simulink model "HQEV_MiL_20160830_integrate_r2017a"  (Simulink 8.9)
settings: Solver=FixedStepDiscrete  StartTime=0.0  StopTime=inf  FixedStep=0.01  RelTol=1e-3  EnableMultiTasking=on
PostLoadFcn:
  | , if any(exist('dsrtsu_mdlpostloadfcn', 'file') == [2, 3, 6]), try dsrtsu_mdlpostloadfcn('Execute', bdroot); catch fprintf('Error in PostLoadFcn (dsrtsu_mdlpostloadfcn) for model "%s":\n %s\n', bdroot, lasterr); end, end,
values from neighbouring files (symbols this model uses):
  Bat_C_Ah = 36    [parameter_V1.mat]
  Bat_ocv_xIndex = [5 10 20 30 40 50 60 70 80 90 95]    [parameter_V1.mat]
  Bat_ocv_z = [329 332 340 345 347 351 358 372 377 386 391]    [parameter_V1.mat]
  Bat_R_ohm_z = [4.41 3.46 1.57 1.07 0.76 0.63 0.55 0.44 0.41 0.4 0.4 3.14 ... (66 elements, 11x6)]    [parameter_V1.mat]
  Bat_SOC_Init = 90    [parameter_V1.mat]
  Env_hum_pct_Ambient = 30    [parameter_V1.mat]
  Env_Slope_deg = 0    [parameter_V1.mat]
  Env_Temp_degC_Ambient = 25    [parameter_V1.mat]
  Env_v_kmph_HWind = 0    [parameter_V1.mat]
  Reducer_F_i = 7.23    [parameter_V1.mat]
  Reducer_R_i = 7.23    [parameter_V1.mat]
  Veh =     [parameter_V1.mat]
  Veh_A_m2_Fr = 2.246    [parameter_V1.mat]
  Veh_F_Brake =     [parameter_V1.mat]
  Veh_fac_AirDrag = 0.326    [parameter_V1.mat]
  Veh_fac_WhDragFrict_0 = 0.011    [parameter_V1.mat]
  Veh_g_mps2_C = 9.81    [parameter_V1.mat]
  Veh_GainBrake =     [parameter_V1.mat]
  Veh_h_m_COGHigh = 0.5    [parameter_V1.mat]
  Veh_J_kgm2_Wh = 1.3635    [parameter_V1.mat]
  Veh_L_m_AxlBas = 2.63    [parameter_V1.mat]
  Veh_M_kg = 1427    [parameter_V1.mat]
  Veh_mu_Brake = 0.4    [parameter_V1.mat]
  Veh_mu_Tyre =     [parameter_V1.mat]
  Veh_num_FrictPair = 8    [parameter_V1.mat]
  Veh_pct_Brk = 70    [parameter_V1.mat]
  Veh_r_dyn =     [parameter_V1.mat]
  Veh_r_m_BrkDisk = 0.136    [parameter_V1.mat]
  Veh_rho_kgpm3_Air = 1.2258    [parameter_V1.mat]
undefined symbols (not defined in the file or in its folder): DiscIntNeverNeededParam, p_bool_False_M, p_bool_True_M
libraries: BaseOperationLib_Browser x38, simulink x8, DTQC_lib x1, ERR_lib x1, MQM_lib x1, PTCL_lib x1, PUD_lib x1, TQD_lib x1, TQR_lib x1, VMM_lib x1, ACCA_lib x1, BBCA_lib x1
(part 5 of 15)

== system HQEV_MiL_20160830_integrate_r2017a/MiL/Test_Integration/ESP/Subsystem/ABS ==
  In1 : Inport
  Bus Selector : BusSelector  OutputSignals=Vehicle.v_Veh
  Bus Selector1 : BusSelector  OutputSignals=Drv.signal1.BrkPed_pct
  Bus Selector2 : BusSelector  OutputSignals=IO.ABS_ErrorStatus,IO.ABS_Intervention,IO.ASR1_ASRErrorStatus,IO.ASR1_ASRIntervention,IO.ESP_ErrorStatus,IO.ESP_Intervention
  Constant{,1..3,10..11} (6 alike) : Constant  Value=0
  Lookup Table : Lookup  InputValues=[0 100]  Table=[0 200]
  Checksum_ABS_1 : Outport
  WheelSpeed_FL : Outport  Port=2
  WheelSpeed_FR : Outport  Port=3
  ABS_VehicleSpeed : Outport  Port=4
  LiveCounter_ABS_1 : Outport  Port=5
  Checksum_ABS_2 : Outport  Port=6
  WheelSpeed_RL : Outport  Port=7
  WheelSpeed_RR : Outport  Port=8
  ABS_MasterCylinderPressure : Outport  Port=9
  LiveCounter_ABS_2 : Outport  Port=10
  ABS_ErrorStatus : Outport  Port=11
  ABS_Intervention : Outport  Port=12
  ASR_ErrorStatus : Outport  Port=13
  ASR_Intervention : Outport  Port=14
  ESP_ErrorStatus : Outport  Port=15
  ESP_Intervention : Outport  Port=16
  HHC_Status : Outport  Port=17
  HHC_Available : Outport  Port=18
  wires:
  Constant/1 -> Checksum_ABS_1/1
  In1/1 -> Bus Selector/1, Bus Selector2/1, Bus Selector1/1
  Bus Selector/1 -> WheelSpeed_FL/1, WheelSpeed_FR/1, ABS_VehicleSpeed/1, WheelSpeed_RL/1, WheelSpeed_RR/1  "<v_Veh>"
  Constant1/1 -> LiveCounter_ABS_1/1
  Constant2/1 -> Checksum_ABS_2/1
  Bus Selector1/1 -> Lookup Table/1  "<BrkPed_pct>"
  Lookup Table/1 -> ABS_MasterCylinderPressure/1
  Constant3/1 -> LiveCounter_ABS_2/1
  Bus Selector2/1 -> ABS_ErrorStatus/1  "<ABS_ErrorStatus>"
  Bus Selector2/2 -> ABS_Intervention/1  "<ABS_Intervention>"
  Bus Selector2/3 -> ASR_ErrorStatus/1  "<ASR1_ASRErrorStatus>"
  Bus Selector2/4 -> ASR_Intervention/1  "<ASR1_ASRIntervention>"
  Bus Selector2/5 -> ESP_ErrorStatus/1  "<ESP_ErrorStatus>"
  Bus Selector2/6 -> ESP_Intervention/1  "<ESP_Intervention>"
  Constant10/1 -> HHC_Status/1
  Constant11/1 -> HHC_Available/1

== system HQEV_MiL_20160830_integrate_r2017a/MiL/Test_Integration/ESP/Subsystem/ASR ==
  In1 : Inport
  Bus Selector2 : BusSelector  OutputSignals=IO.ASR_TorqueReductionFast,IO.MSR_TorqueIncrease,IO.ASR_StatusTRFast,IO.MSR_StatusTI
  Constant : Constant  Value=0
  Constant3 : Constant  Value=0
  Checksum_ASR_1 : Outport
  ASR_TorqueReductionFast : Outport  Port=2
  MSR_TorqueIncrease : Outport  Port=3
  LiveCounter_ASR_1 : Outport  Port=4
  ASR_StatusTRFast : Outport  Port=5
  MSR_StatusTI : Outport  Port=6
  wires:
  In1/1 -> Bus Selector2/1
  Constant/1 -> Checksum_ASR_1/1
  Bus Selector2/1 -> ASR_TorqueReductionFast/1  "<ASR_TorqueReductionFast>"
  Bus Selector2/2 -> MSR_TorqueIncrease/1  "<MSR_TorqueIncrease>"
  Constant3/1 -> LiveCounter_ASR_1/1
  Bus Selector2/3 -> ASR_StatusTRFast/1  "<ASR_StatusTRFast>"
  Bus Selector2/4 -> MSR_StatusTI/1  "<MSR_StatusTI>"

== system HQEV_MiL_20160830_integrate_r2017a/MiL/Test_Integration/ESP/Subsystem/ASR2 ==
  In1 : Inport
  Bus Selector51 : BusSelector  OutputSignals=IO
  Bus Selector52 : BusSelector  OutputSignals=ASR2TrqRdctFastASR2,ASR2TrqIncrsMSR2,ASR2StTRFastASR2,ASR2StTIMSR2,ABS6RegenTrqReq,ABS6StRegenTrqReq
  ASR2TrqRdctFastASR2 : Outport
  ASR2TrqIncrsMSR2 : Outport  Port=2
  ASR2StTRFastASR2 : Outport  Port=3
  ASR2StTIMSR2 : Outport  Port=4
  ABS6RegenTrqReq : Outport  Port=5
  ABS6StRegenTrqReq : Outport  Port=6
  wires:
  Bus Selector51/1 -> Bus Selector52/1  "<IO>"
  In1/1 -> Bus Selector51/1
  Bus Selector52/1 -> ASR2TrqRdctFastASR2/1  "<ASR2TrqRdctFastASR2>"
  Bus Selector52/2 -> ASR2TrqIncrsMSR2/1  "<ASR2TrqIncrsMSR2>"
  Bus Selector52/3 -> ASR2StTRFastASR2/1  "<ASR2StTRFastASR2>"
  Bus Selector52/4 -> ASR2StTIMSR2/1  "<ASR2StTIMSR2>"
  Bus Selector52/5 -> ABS6RegenTrqReq/1  "<ABS6RegenTrqReq>"
  Bus Selector52/6 -> ABS6StRegenTrqReq/1  "<ABS6StRegenTrqReq>"

== system HQEV_MiL_20160830_integrate_r2017a/MiL/Test_Integration/ESP/Subsystem/EPB ==
  In1 : Inport
  Constant{,1..3} (4 alike) : Constant  Value=0
  Terminator : Terminator
  Checksum_EPB_1 : Outport
  LiveCounter_EPB_1 : Outport  Port=2
  EPB_Status : Outport  Port=3
  EPB_ErrorStatus : Outport  Port=4
  wires:
  Constant/1 -> Checksum_EPB_1/1
  Constant1/1 -> LiveCounter_EPB_1/1
  Constant2/1 -> EPB_Status/1
  Constant3/1 -> EPB_ErrorStatus/1
  In1/1 -> Terminator/1

== system HQEV_MiL_20160830_integrate_r2017a/MiL/Test_Integration/ESP/Subsystem/YRS ==
  In1 : Inport
  Bus Selector : BusSelector  OutputSignals=Vehicle.acc
  Constant{,1..8} (9 alike) : Constant  Value=0
  Checksum_YRS_1 : Outport
  AX1 : Outport  Port=2
  AY1 : Outport  Port=3
  LiveCounter_YRS_1 : Outport  Port=4
  YRSStatus : Outport  Port=5
  YRSErrorStatus : Outport  Port=6
  Checksum_YRS2 : Outport  Port=7
  AX1Offset : Outport  Port=8
  AY1Offset : Outport  Port=9
  LiveCounter_YRS2 : Outport  Port=10
  wires:
  In1/1 -> Bus Selector/1
  Constant/1 -> Checksum_YRS_1/1
  Bus Selector/1 -> AX1/1  "<acc>"
  Constant1/1 -> AY1/1
  Constant2/1 -> LiveCounter_YRS_1/1
  Constant3/1 -> YRSStatus/1
  Constant4/1 -> YRSErrorStatus/1
  Constant5/1 -> Checksum_YRS2/1
  Constant6/1 -> AX1Offset/1
  Constant7/1 -> AY1Offset/1
  Constant8/1 -> LiveCounter_YRS2/1

== system HQEV_MiL_20160830_integrate_r2017a/MiL/Test_Integration/Epark/Subsystem/Epark ==
  In1 : Inport
  Epark_Process : Subsystem
  Subsystem : Subsystem
  Subsystem1 : Subsystem
  Subsystem2 : Subsystem
  Subsystem3 : Subsystem
  Subsystem4 : Subsystem
  Subsystem5 : Subsystem
  Subsystem6 : Subsystem
  ePARK_MOTOR_OPEN_CKT : Outport
  ePARK_MOTOR_JAMMED_PARK : Outport  Port=2
  ePARK_MOTOR_JAMMED_UNPARK : Outport  Port=3
  ePARK_MOTOR_JAMMED_MIDDL : Outport  Port=4
  ePARK_HALL_SENSOR_INVALID : Outport  Port=5
  ePARK_LOST_COMM_VCU : Outport  Port=6
  ePARK_CAN_ERR : Outport  Port=7
  ParkLock : Outport  Port=8
  ParkSensor : Outport  Port=9
  DriveSensor : Outport  Port=10
  wires:
  Subsystem/1(ePARK_MOTOR_OPEN_CKT) -> ePARK_MOTOR_OPEN_CKT/1
  Subsystem1/1(ePARK_MOTOR_JAMMED_PARK) -> ePARK_MOTOR_JAMMED_PARK/1
  Subsystem3/1(ePARK_MOTOR_JAMMED_MIDDL) -> ePARK_MOTOR_JAMMED_MIDDL/1
  Subsystem4/1(ePARK_HALL_SENSOR_INVALID) -> ePARK_HALL_SENSOR_INVALID/1
  Subsystem5/1(ePARK_LOST_COMM_VCU) -> ePARK_LOST_COMM_VCU/1
  Subsystem6/1(ePARK_CAN_ERR) -> ePARK_CAN_ERR/1
  Subsystem2/1(ePARK_MOTOR_JAMMED_UNPARK) -> ePARK_MOTOR_JAMMED_UNPARK/1
  In1/1 -> Epark_Process/1(In3)
  Epark_Process/1(ParkLock) -> ParkLock/1
  Epark_Process/2(ParkSensor) -> ParkSensor/1
  Epark_Process/3(DriveSensor) -> DriveSensor/1

== system HQEV_MiL_20160830_integrate_r2017a/MiL/Test_Integration/HCU/HCU/AccPedpct2mV ==
  In1 : Inport
  Add : Sum
  Constant8 : Constant  Value=29.25
  Constant9 : Constant  Value=1100
  Gain : Gain  Gain=0.5
  Product1 : Product  RndMeth=Zero
  Out1 : Outport
  Out2 : Outport  Port=2
  wires:
  Gain/1 -> Out2/1
  Constant9/1 -> Add/2
  Product1/1 -> Add/1
  Constant8/1 -> Product1/2
  In1/1 -> Product1/1
  Add/1 -> Out1/1, Gain/1
